simulink model "My_project_2"  (R2023b)
settings: Solver=VariableStepAuto  StartTime=0.0  StopTime=3  MaxStep=1e-6  RelTol=1e-3
libraries: spsThyristorLib x4, spsVoltageMeasurementLib x3, spsSeriesRLCBranchLib x2, spspowerguiLib x2, spsACVoltageSourceLib x1, dspswit3 x1, spsUniversalBridgeLib x1
settings Model: Creator=hp  LastModifiedBy=hp

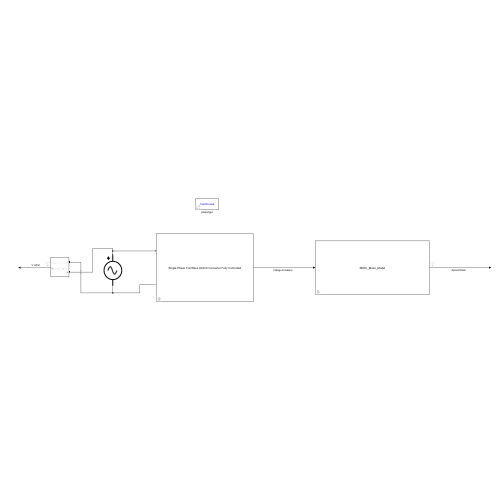
[thumbnail: Simulink's stored preview of the top-level diagram]
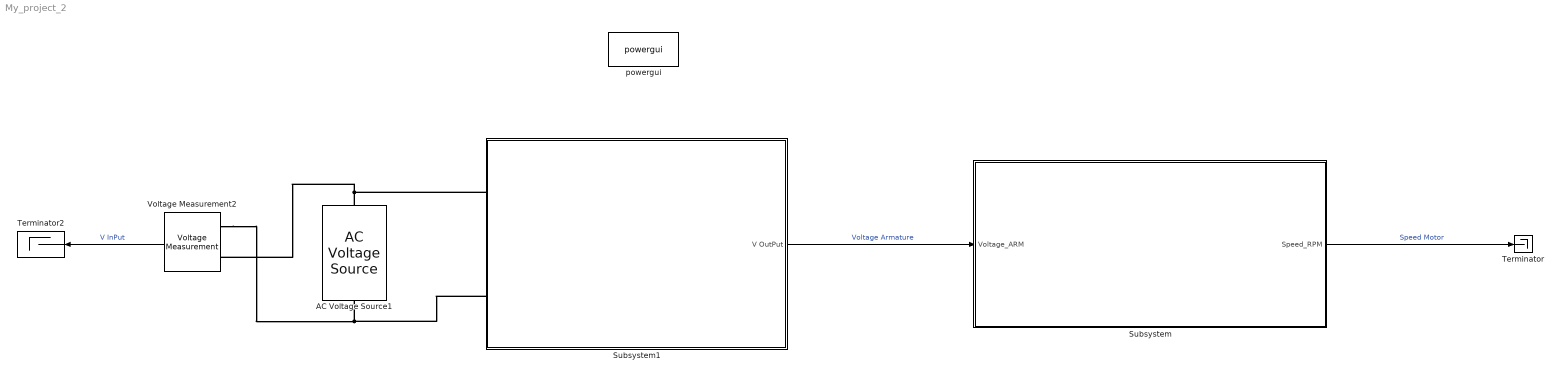
== system My_project_2 ==
  AC Voltage Source1 : spsACVoltageSourceLib/AC Voltage Source  Amplitude=240*sqrt(2)  Phase=0  Frequency=50  SampleTime=0  Measurements=None  BusType=swing  Pref=10e3  Qref=0  Qmin=-inf  Qmax=+inf
  Subsystem : Subsystem  mask{Ra=2.581, La=0.0281, Kf=1.25, J=0.0221, B=0.002953, TL=5}
      mask prompts: Ra "Armature Resistance"; La "Armature Inductance"; Kf "Constant"; J "Moment inertia"; B "Damping Coefficient"; TL "Load Torque"
      mask DialogControl DescGroupVar Prompt: Separately Exited Dc Motor
      mask DialogControl DescTextVar Prompt: This model reprsent to separately exited dc motor
      mask DialogControl Parameters Prompt: Parameters of model
      mask Display: disp(['SEDC_Motor_Model']);
  Subsystem1 : Subsystem
      mask Display: disp('Single Phase Full Wave AC/DC Converter Fully Controlled');
  Terminator : Terminator
  Terminator2 : Terminator
  Voltage Measurement2 : spsVoltageMeasurementLib/Voltage Measurement  PhasorSimulation=off  OutputType=Complex  PSBequivalent=0
  powergui : spspowerguiLib/powergui  Priority=1  SimulationMode=Continuous  SampleTime=50e-6  frequency=60  Iterations=50  frequencyindice=50  Pbase=100e6  ErrMax=1e-4  UnitsV=kV  UnitsW=MW  buscounter=0  FunctionMessages=off  echomessages=off  EnableUseOfTLC=off  CurrentSourceSwitches=off  DisableSnubberDevices=off  DisableRonSwitches=off  DisableVfSwitches=off  DisplayEquations=off  AutomaticDiscreteSolvers=off  SolverType=Tustin/Backward Euler (TBE)  Interpol=off  ExternalGateDelay=off  methode=off  Ts=100  x0status=blocks  SPID=on  SwTol=0  HookPort=off  NonlinearTolerance=1e-4  nMaxIteration=100  ContinueOnMaxIteration=off  RestoreLinks=warning  ResistiveCurrentMeasurement=off  Frange=[0:2:500]  Ylog=off  Xlog=on  ShowGrid=off  save=off  variable=ZData  structure=0  ZoomFFT=off  StartTime=0.0  cycles=1  DisplayStyle=1  fundamental=60  FreqAxis=off  MaxFrequency=1000  frequencyindicesteady=1  RmsSteady=1  display=off
  wires:
  Subsystem/1(Speed_RPM) -> Terminator/1  "Speed Motor"
  Voltage Measurement2/1 -> Terminator2/1  "V InPut"
  Subsystem1/1(V OutPut) -> Subsystem/1(Voltage_ARM)  "Voltage Armature"
  connections:
  AC Voltage Source1/RConn1 -- Voltage Measurement2/LConn1 -- Subsystem1/LConn1
  Voltage Measurement2/LConn2 -- Subsystem1/LConn2 -- AC Voltage Source1/LConn1

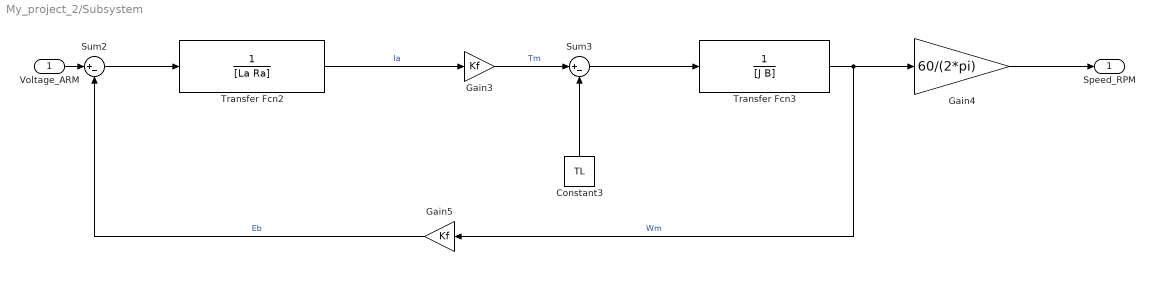
== system My_project_2/Subsystem ==
  Voltage_ARM : Inport
  Constant3 : Constant  Value=TL
  Gain3 : Gain  Gain=Kf
  Gain4 : Gain  Gain=60/(2*pi)
  Gain5 : Gain  Gain=Kf
  Sum2 : Sum  Inputs=|+-
  Sum3 : Sum  Inputs=|+-
  Transfer Fcn2 : TransferFcn  Denominator=[La Ra]
  Transfer Fcn3 : TransferFcn  Denominator=[J B]
  Speed_RPM : Outport
  wires:
  Gain5/1 -> Sum2/2  "Eb"
  Constant3/1 -> Sum3/2
  Gain3/1 -> Sum3/1  "Tm"
  Voltage_ARM/1 -> Sum2/1
  Transfer Fcn2/1 -> Gain3/1  "Ia"
  Transfer Fcn3/1 -> Gain5/1, Gain4/1  "Wm"
  Sum3/1 -> Transfer Fcn3/1
  Sum2/1 -> Transfer Fcn2/1
  Gain4/1 -> Speed_RPM/1

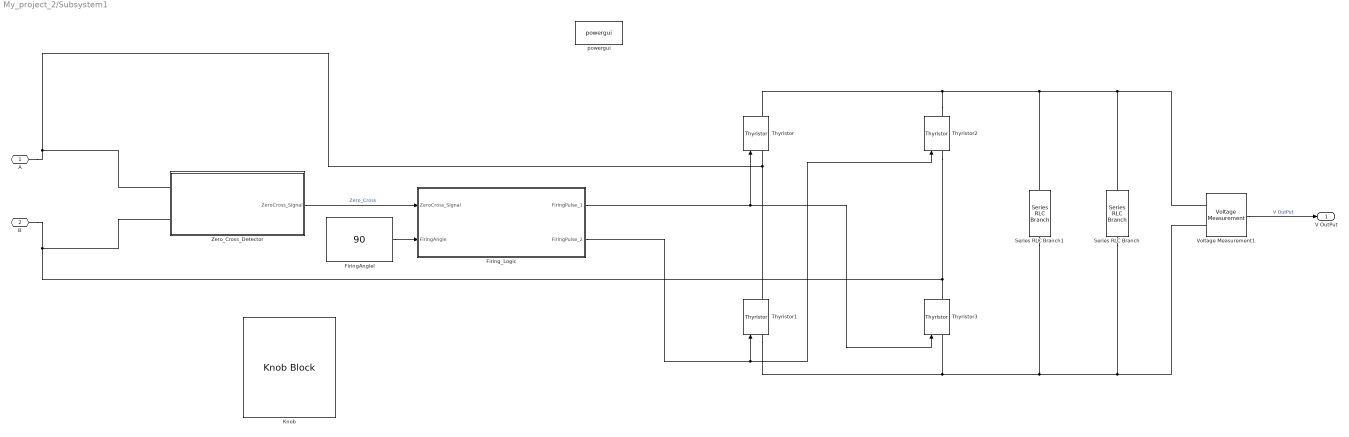
== system My_project_2/Subsystem1 ==
  FiringAnglel : Constant  Value=90
  Firing_Logic : Subsystem
  Knob : KnobBlock  ScaleMax=180
  Series RLC Branch : spsSeriesRLCBranchLib/Series RLC Branch  LConnTagsString=__new0  RConnTagsString=__new0  BranchType=R  Resistance=10*2.581  Inductance=1e-3  SetiL0=off  InitialCurrent=0  Capacitance=1e-6  Setx0=off  InitialVoltage=0  Measurements=None
  Series RLC Branch1 : spsSeriesRLCBranchLib/Series RLC Branch  LConnTagsString=__new0  RConnTagsString=__new0  BranchType=C  Resistance=50  Inductance=1e-3  SetiL0=off  InitialCurrent=0  Capacitance=10000*10^-6  Setx0=off  InitialVoltage=0  Measurements=None
  Thyristor{,1..3} (4 alike) : spsThyristorLib/Thyristor  Ron=0.001  Lon=0  Vf=0.8  IC=0  Rs=500  Cs=250e-9  Measurements=on
  Voltage Measurement1 : spsVoltageMeasurementLib/Voltage Measurement  PhasorSimulation=off  OutputType=Complex  PSBequivalent=0
  Zero_Cross_Detector : Subsystem
  powergui : spspowerguiLib/powergui  Priority=1  SimulationMode=Continuous  SampleTime=50e-6  frequency=60  Iterations=50  frequencyindice=50  Pbase=100e6  ErrMax=1e-4  UnitsV=kV  UnitsW=MW  buscounter=0  FunctionMessages=off  echomessages=off  EnableUseOfTLC=off  CurrentSourceSwitches=off  DisableSnubberDevices=off  DisableRonSwitches=off  DisableVfSwitches=off  DisplayEquations=off  AutomaticDiscreteSolvers=off  SolverType=Tustin/Backward Euler (TBE)  Interpol=off  ExternalGateDelay=off  methode=off  Ts=100  x0status=blocks  SPID=on  SwTol=0  HookPort=off  NonlinearTolerance=1e-4  nMaxIteration=100  ContinueOnMaxIteration=off  RestoreLinks=warning  ResistiveCurrentMeasurement=off  Frange=[0:2:500]  Ylog=off  Xlog=on  ShowGrid=off  save=off  variable=ZData  structure=0  ZoomFFT=off  StartTime=0.0  cycles=1  DisplayStyle=1  fundamental=60  FreqAxis=off  MaxFrequency=1000  frequencyindicesteady=1  RmsSteady=1  display=off
  A : PMIOPort  Side=Left
  B : PMIOPort  Port=2  Side=Left
  V OutPut : Outport
  wires:
  Firing_Logic/2(FiringPulse_2) -> Thyristor2/1, Thyristor1/1
  Voltage Measurement1/1 -> V OutPut/1  "V OutPut"
  Firing_Logic/1(FiringPulse_1) -> Thyristor3/1, Thyristor/1
  FiringAnglel/1 -> Firing_Logic/2(FiringAngle)
  Zero_Cross_Detector/1(ZeroCross_Signal) -> Firing_Logic/1(ZeroCross_Signal)  "Zero_Cross"
  connections:
  Thyristor/LConn1 -- Thyristor1/RConn1 -- A/RConn1 -- Zero_Cross_Detector/LConn1
  Zero_Cross_Detector/LConn2 -- B/RConn1 -- Thyristor3/RConn1 -- Thyristor2/LConn1
  Thyristor2/RConn1 -- Series RLC Branch1/LConn1 -- Voltage Measurement1/LConn1 -- Series RLC Branch/LConn1 -- Thyristor/RConn1
  Thyristor3/LConn1 -- Thyristor1/LConn1 -- Series RLC Branch/RConn1 -- Voltage Measurement1/LConn2 -- Series RLC Branch1/RConn1

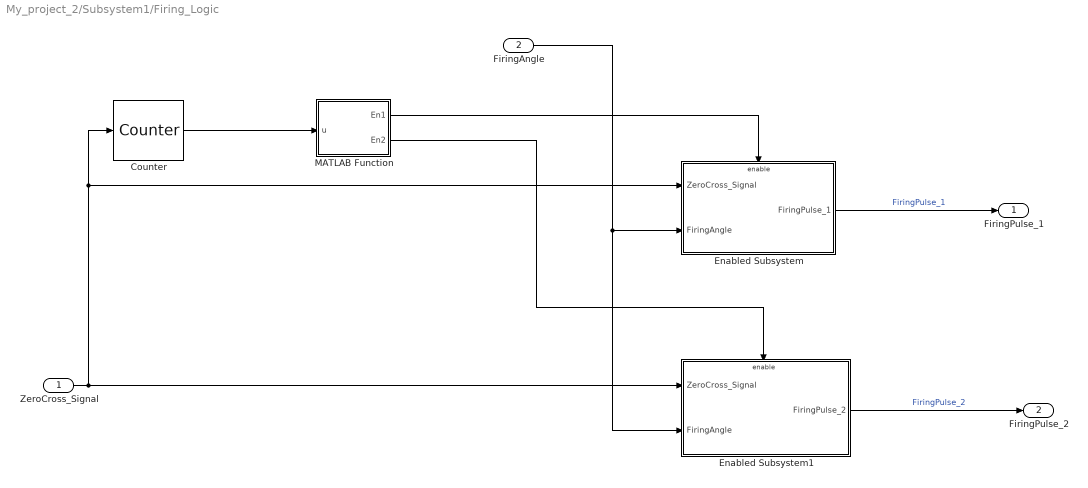
== system My_project_2/Subsystem1/Firing_Logic ==
  ZeroCross_Signal : Inport
  FiringAngle : Inport  Port=2
  Counter : dspswit3/Counter  Direction=Up  CountEvent=Rising edge  CounterSize=User defined  MaxCount=255  InitialCount=0  Output=Count  HitValue=32  ResetInput=off  SamplesPerFrame=1  Ts=1  CntDtype=double  HitDtype=Logical
  Enabled Subsystem : Subsystem  TreatAsAtomicUnit=on
  Enabled Subsystem1 : Subsystem  TreatAsAtomicUnit=on
  MATLAB Function : MATLAB Function  TreatAsAtomicUnit=on
  FiringPulse_1 : Outport
  FiringPulse_2 : Outport  Port=2
  wires:
  ZeroCross_Signal/1 -> Enabled Subsystem1/1(ZeroCross_Signal), Counter/1, Enabled Subsystem/1(ZeroCross_Signal)
  Counter/1 -> MATLAB Function/1(u)
  MATLAB Function/2(En2) -> Enabled Subsystem1/Enable
  FiringAngle/1 -> Enabled Subsystem/2(FiringAngle), Enabled Subsystem1/2(FiringAngle)
  Enabled Subsystem/1(FiringPulse_1) -> FiringPulse_1/1  "FiringPulse_1"
  Enabled Subsystem1/1(FiringPulse_2) -> FiringPulse_2/1  "FiringPulse_2"
  MATLAB Function/1(En1) -> Enabled Subsystem/Enable

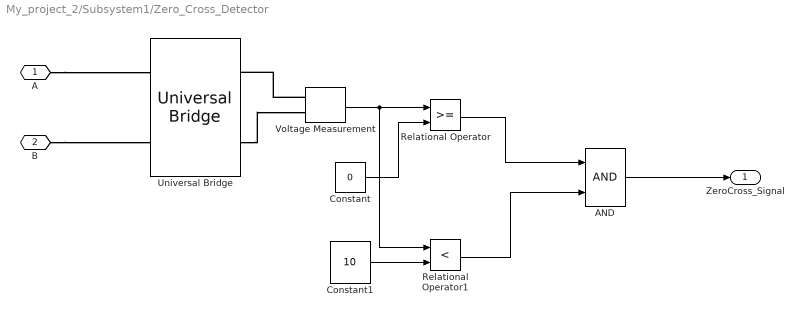
== system My_project_2/Subsystem1/Zero_Cross_Detector ==
  AND : Logic  AllPortsSameDT=off  OutDataTypeStr=boolean
  Constant : Constant  Value=0
  Constant1 : Constant  Value=10
  Relational Operator : RelationalOperator  OutDataTypeStr=boolean  RndMeth=Simplest  InputSameDT=off
  Relational Operator1 : RelationalOperator  Operator=<  OutDataTypeStr=boolean  RndMeth=Simplest  InputSameDT=off
  Universal Bridge : spsUniversalBridgeLib/Universal Bridge  Arms=2  SnubberResistance=1e5  SnubberCapacitance=inf  Device=Diodes  Ron=1e-3  Lon=0  ForwardVoltages="[  0  0  ]"  ForwardVoltage=0  GTOparameters=[ 10e-6 , 20e-6 ]  IGBTparameters=[ 1e-6 , 2e-6 ]  Measurements=None  Measurements_2=None  converterType=Rectifier
  Voltage Measurement : spsVoltageMeasurementLib/Voltage Measurement  PhasorSimulation=off  OutputType=Complex  PSBequivalent=0
  A : PMIOPort  Side=Left
  B : PMIOPort  Port=2  Side=Left
  ZeroCross_Signal : Outport
  wires:
  AND/1 -> ZeroCross_Signal/1
  Relational Operator1/1 -> AND/2
  Relational Operator/1 -> AND/1
  Constant1/1 -> Relational Operator1/2
  Constant/1 -> Relational Operator/2
  Voltage Measurement/1 -> Relational Operator/1, Relational Operator1/1
  connections:
  Universal Bridge/RConn2 -- Voltage Measurement/LConn2
  Voltage Measurement/LConn1 -- Universal Bridge/RConn1
  A/RConn1 -- Universal Bridge/LConn1
  B/RConn1 -- Universal Bridge/LConn2

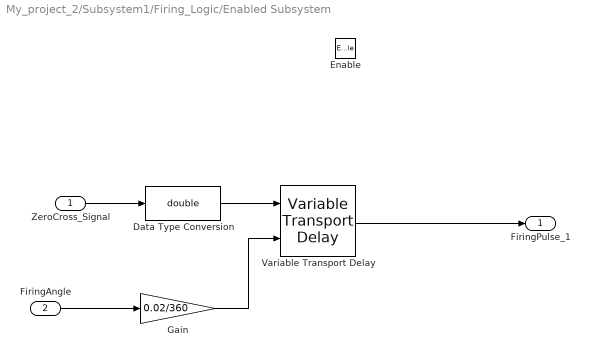
== system My_project_2/Subsystem1/Firing_Logic/Enabled Subsystem ==
  ZeroCross_Signal : Inport
  FiringAngle : Inport  Port=2
  Enable : EnablePort
  Data Type Conversion : DataTypeConversion  OutDataTypeStr=double  SaturateOnIntegerOverflow=off  RndMeth=Floor
  Gain : Gain  Gain=0.02/360
  Variable Transport Delay : VariableTransportDelay  MaximumDelay=10
  FiringPulse_1 : Outport
  wires:
  FiringAngle/1 -> Gain/1
  Gain/1 -> Variable Transport Delay/2
  Variable Transport Delay/1 -> FiringPulse_1/1
  ZeroCross_Signal/1 -> Data Type Conversion/1
  Data Type Conversion/1 -> Variable Transport Delay/1

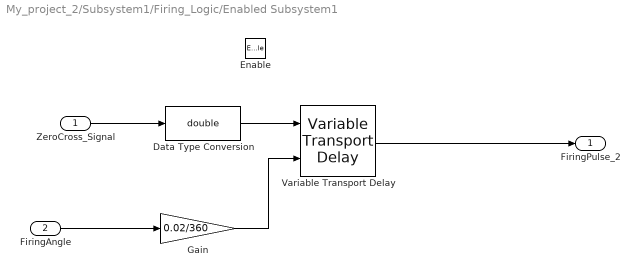
== system My_project_2/Subsystem1/Firing_Logic/Enabled Subsystem1 ==
  ZeroCross_Signal : Inport
  FiringAngle : Inport  Port=2
  Enable : EnablePort
  Data Type Conversion : DataTypeConversion  OutDataTypeStr=double  SaturateOnIntegerOverflow=off  RndMeth=Floor
  Gain : Gain  Gain=0.02/360
  Variable Transport Delay : VariableTransportDelay  MaximumDelay=10
  FiringPulse_2 : Outport
  wires:
  Variable Transport Delay/1 -> FiringPulse_2/1
  FiringAngle/1 -> Gain/1
  ZeroCross_Signal/1 -> Data Type Conversion/1
  Data Type Conversion/1 -> Variable Transport Delay/1
  Gain/1 -> Variable Transport Delay/2

== matlab function My_project_2/Subsystem1/Firing_Logic/MATLAB Function ==
  data: u input; En1 output; En2 output
function [En1 , En2] = fcn(u)
En1 = 0;
En2 = 0;

if mod (u,2) == 0
    En1 = 1;
    En2 = 0;
end

if mod (u,2) == 1
    En1 = 0;
    En2 = 1;
end
